simulink model "Pitoni_0"  (R2023a)
settings: Solver=VariableStepAuto  StartTime=0.0  StopTime=10  RelTol=1e-3
(part 2 of 2)

== matlab function Pitoni_0/media ==
  data: u input; y output
function y = media(u)

y = mean(u);

== matlab function Pitoni_0/media2 ==
  data: u input; y output
function y = media(u)

y = mean(u);

== matlab function Pitoni_0/media3 ==
  data: u input; y output
function y = media(u)

y = mean(u);

== matlab function Pitoni_0/media4 ==
  data: u input; y output
function y = media(u)

y = mean(u);

== matlab function Pitoni_0/media1 ==
  data: u input; y output
function y = media(u)

y = mean(u);
